simulink model "Practica6"  (R2023a)
settings: Solver=VariableStepAuto  StartTime=0.0  StopTime=0.05  RelTol=1e-3
values from neighbouring files (symbols this model uses):
  C = 10e-6    (= 1e-05)    [Practica5gf.m]
  L = 2e-3    (= 0.002)    [Practica5gf.m]
  R = 10    [Practica5gf.m]
settings Model: Creator=mluser  LastModifiedBy=mluser

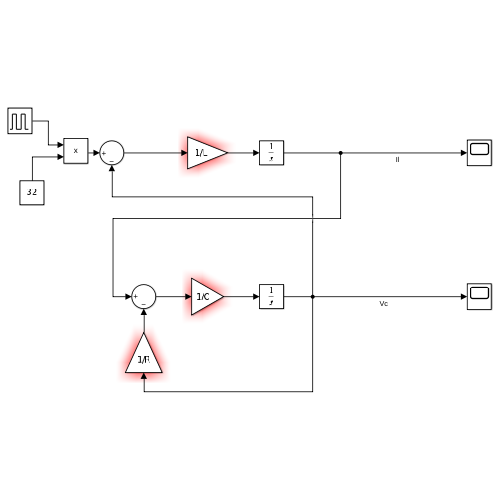
[thumbnail: Simulink's stored preview of the top-level diagram]
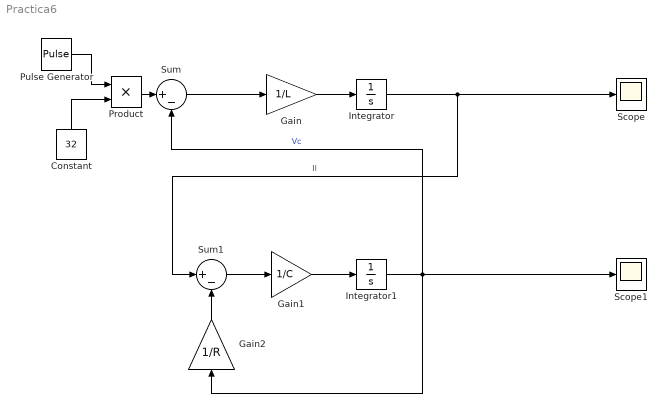
== system Practica6 ==
  Constant : Constant  Value=32
  Gain : Gain  Gain=1/L
  Gain1 : Gain  Gain=1/C
  Gain2 : Gain  Gain=1/R
  Integrator : Integrator
  Integrator1 : Integrator
  Product : Product
  Pulse Generator : DiscretePulseGenerator  PulseType=Time based  Period=1/100000  PulseWidth=40
  Scope : Scope
  Scope1 : Scope
  Sum : Sum  Inputs=|+-
  Sum1 : Sum  Inputs=|+-
  wires:
  Sum/1 -> Gain/1
  Gain/1 -> Integrator/1
  Integrator/1 -> Sum1/1, Scope/1  "Il"
  Gain1/1 -> Integrator1/1
  Sum1/1 -> Gain1/1
  Integrator1/1 -> Gain2/1, Scope1/1, Sum/2  "Vc"
  Product/1 -> Sum/1
  Pulse Generator/1 -> Product/1
  Constant/1 -> Product/2
  Gain2/1 -> Sum1/2
